simulink model "mpc_model_dual_module_tobecombined"  (R2019a)
settings: Solver=FixedStepAuto  StartTime=0.0  StopTime=Tfinal  RelTol=1e-3
values from neighbouring files (symbols this model uses):
  A = [-0.0285 -0.0014; -0.0371 -0.1476]    [model.m]
  DCLINK_Cap = 1000e-12    (= 1e-09)    [mpc_model_parameters.m]    (also in mpc_model_parameters_dual_module.m = 0.001)
  FluxPM = MeanInducedVoltagePeak/(2*pi*100)    [mpc_model_parameters.m]    (also in mpc_model_parameters_dual_module.m)
  Inertia = 1e-2    (= 0.01)    [mpc_model_parameters.m]    (also in mpc_model_parameters_dual_module.m)
  iqrated = Trated/(1.5*PolePairs*FluxPM)    [mpc_model_parameters.m]    (also in mpc_model_parameters_dual_module.m)
  Ls = 3.5e-3    (= 0.0035)    [MPC_id_iq.m]    (also in mpc_model_parameters.m = 0.00351; mpc_model_parameters_dual_module.m = 0.00343)
  M1_FaultTime = 0.25    [mpc_model_parameters_dual_module.m]
  M2_FaultTime = 20    [mpc_model_parameters_dual_module.m]
  MeanLd = (1/12)*(Module1Phase_A_Ld+Module1Phase_B_Ld+Module1Phase_C_Ld+     Module2Phase_A_Ld+Module2Phase_B_Ld+Module2Phase_C_Ld+     Module3Phase_A_Ld+Module3Phase_B_Ld+Module3Phase_C_Ld+     Module4Phase_A_Ld+Module4Phase_B_Ld+Module4Phase_C_Ld)    [mpc_model_parameters.m]    (also in mpc_model_parameters_dual_module.m)
  MeanLq = (1/12)*(Module1Phase_A_Lq+Module1Phase_B_Lq+Module1Phase_C_Lq+     Module2Phase_A_Lq+Module2Phase_B_Lq+Module2Phase_C_Lq+     Module3Phase_A_Lq+Module3Phase_B_Lq+Module3Phase_C_Lq+     Module4Phase_A_Lq+Module4Phase_B_Lq+Module4Phase_C_Lq)    [mpc_model_parameters.m]    (also in mpc_model_parameters_dual_module.m)
  PolePairs = 10    [mpc_model_parameters.m]    (also in mpc_model_parameters_dual_module.m)
  Rin = 1e-3    (= 0.001)    [mpc_model_parameters.m]    (also in mpc_model_parameters_dual_module.m)
  Rs = 0.531    [Loss_Distribution.m]    (also in MPC_id_iq.m; mpc_model_parameters.m = 0.321; mpc_model_parameters_dual_module.m = 0.539)
  Sampling_time = 1e-6    (= 1e-06)    [mpc_model_parameters.m]    (also in mpc_model_parameters_dual_module.m)
  SpeedRef1 = 50    [mpc_model_parameters.m]    (also in mpc_model_parameters_dual_module.m = 35)
  SpeedRef2 = 100    [mpc_model_parameters.m]    (also in mpc_model_parameters_dual_module.m = 35)
  SpeedRefUpdateTime = 0.25    [mpc_model_parameters.m]    (also in mpc_model_parameters_dual_module.m = 1.75)
  Tload1 = 5    [mpc_model_parameters.m]    (also in mpc_model_parameters_dual_module.m = 30)
  Tload2 = 10    [mpc_model_parameters.m]    (also in mpc_model_parameters_dual_module.m = 63.6619772368)
  TloadUpdateTime = 0.5    [mpc_model_parameters.m]    (also in mpc_model_parameters_dual_module.m)
  Vdc = 50    [mpc_model_parameters.m]    (also in mpc_model_parameters_dual_module.m = 40)
  Vin = Vdc + Rin*(Pout/Vdc)    (= 50.04)    [mpc_model_parameters.m]    (also in mpc_model_parameters_dual_module.m = 40.05)
  ViscousFriction = 1e-3    (= 0.001)    [mpc_model_parameters.m]    (also in mpc_model_parameters_dual_module.m)
undefined symbols (not defined in the file or in its folder): DiscIntNeverNeededParam
libraries: powerlib x24, dspswit3 x13, fl_lib x5, simulink x3, powerlib_meascontrol x3, nesl_utility x3, sdl_lib x1, dspsigops x1
(part 1 of 2)
settings Model: Creator=hakan  LastModifiedBy=hakan
settings SolverCC: ZeroCrossAlgorithm=Adaptive
settings DebuggingCC: IgnoredZcDiagnostic=none

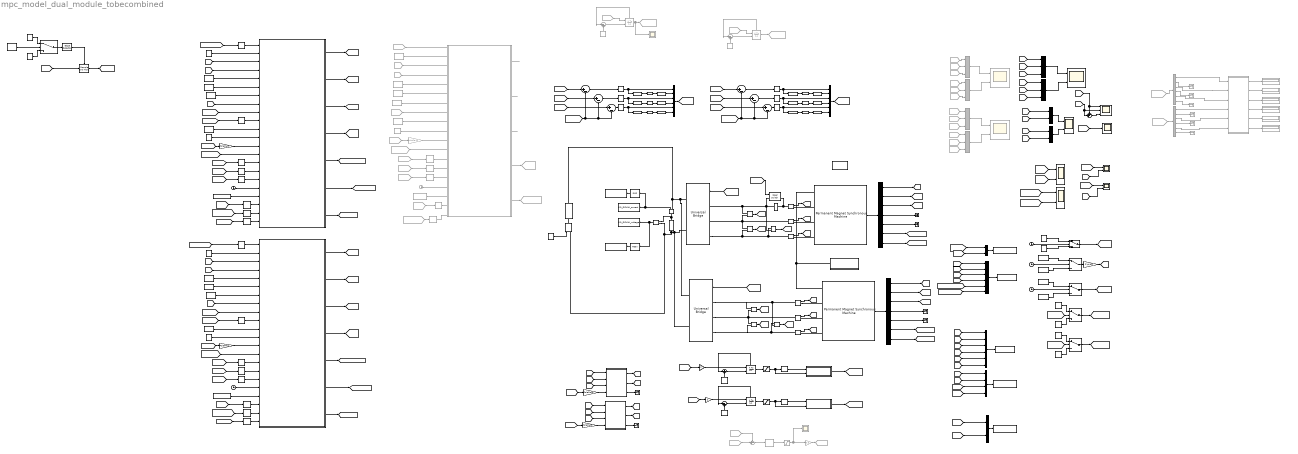
== system mpc_model_dual_module_tobecombined ==
  note: M1_thetam & M2_thetam will be the but they are seperated anyway
  A_DCLINK_current : ToWorkspace  VariableName=M1_DCLINK_current  SaveFormat=Structure With Time  SampleTime=-1
  A_DCLINK_current_rms : ToWorkspace  VariableName=M1_DCLINK_current_rms  SaveFormat=Structure With Time  SampleTime=-1
  A_DCLINK_voltage : ToWorkspace  VariableName=M1_DCLINK_voltage  SaveFormat=Structure With Time  SampleTime=-1
  A_DCLINK_voltage_mean : ToWorkspace  VariableName=M1_DCLINK_voltage_mean  SaveFormat=Structure With Time  SampleTime=-1
  Bus Creator : BusCreator  Inputs=6
  Bus Creator1 : BusCreator  Inputs=6
  Bus Creator{3,10..12} (4 alike) : BusCreator  Inputs=2
  Bus Creator2 : BusCreator  Inputs=4
  Bus Creator{4..7} (4 alike) : BusCreator  Commented=on  Inputs=3
  Bus Creator8 : BusCreator  Inputs=3
  Bus Creator9 : BusCreator  Inputs=3
  Bus Selector : BusSelector  OutputSignals=Electromagnetic torque Te (N*m),Rotor speed wm (rad/s),Rotor angle thetam (rad),Stator current is_q (A),Stator current is_d (A),Stator voltage Vs_q (V),Stator voltage Vs_d (V)
  Bus Selector1 : BusSelector  OutputSignals=Electromagnetic torque Te (N*m),Rotor speed wm (rad/s),Rotor angle thetam (rad),Stator current is_q (A),Stator current is_d (A),Stator voltage Vs_q (V),Stator voltage Vs_d (V)
  Clock{,1..2,4..5} (5 alike) : Clock
  Clock3 : Clock  Commented=on
  Compare To Zero : simulink/Logic and Bit Operations/Compare To Zero  relop===  OutDataTypeStr=boolean
  Compare To Zero1 : simulink/Logic and Bit Operations/Compare To Zero  relop===  OutDataTypeStr=boolean
  Constant : Constant  Value=Vin
  Constant1 : Constant  Commented=on  Value=1.04
  Constant10 : Constant  Value=SpeedRef1
  Constant11 : Constant  Value=SpeedRef2
  Constant12 : Constant  Value=Tload2
  Constant13 : Constant  Value=M2_FaultTime
  Constant14 : Constant  Value=Ls
  Constant{4,15,22,27,29,36} (6 alike) : Constant  Value=0
  Constant{16,23,30,37} (4 alike) : Constant
  Constant17 : Constant  Commented=on  Value=M1_FaultTime
  Constant18 : Constant  Value=Rs
  Constant19 : Constant  Value=PolePairs
  Constant2 : Constant  Commented=on  Value=0
  Constant20 : Constant  Value=FluxPM
  Constant21 : Constant  Value=Vdc
  Constant24 : Constant  Value=1.02
  Constant25 : Constant  Value=1.02
  Constant26 : Constant  Commented=on  Value=1.04
  Constant28 : Constant  Value=M1_FaultTime
  Constant3 : Constant  Commented=on  Value=Ls
  Constant31 : Constant  Value=Ls
  Constant32 : Constant  Value=Rs
  Constant33 : Constant  Value=PolePairs
  Constant34 : Constant  Value=FluxPM
  Constant35 : Constant  Value=Vdc
  Constant5 : Constant  Commented=on  Value=Rs
  Constant6 : Constant  Commented=on  Value=PolePairs
  Constant7 : Constant  Commented=on  Value=FluxPM
  Constant8 : Constant  Value=Tload1
  Constant9 : Constant  Commented=on  Value=Vdc
  Controlled Voltage Source : powerlib/Electrical Sources/Controlled Voltage Source  Initialize=on  Source_Type=DC  Amplitude=0  Phase=0  Frequency=0  Measurements=None
      settings: SourceProductName=Simscape Electrical
  Current Measurement{,1..6} (7 alike) : powerlib/Measurements/Current Measurement  PhasorSimulation=off  OutputType=Complex  PSBequivalent=0
      settings: SourceProductName=Simscape Electrical
  DCLINK_Cap : powerlib/Elements/Series RLC Branch  LConnTagsString=__new0  RConnTagsString=__new0  BranchType=C  Resistance=1  Inductance=1e-3  SetiL0=off  InitialCurrent=0  Capacitance=DCLINK_Cap  Setx0=on  InitialVoltage=Vin  Measurements=None
      settings: SourceProductName=Simscape Electrical
  Data Type Conversion{1,3,5,12,14,16} (6 alike) : DataTypeConversion  OutDataTypeStr=boolean
  Data Type Conversion{2,4,6,13,15,17} (6 alike) : DataTypeConversion  OutDataTypeStr=double
  Delay{,2..10,15..20} (16 alike) : Delay  DelayLength=1
  Delay{1,11..14} (5 alike) : Delay  Commented=on  DelayLength=1
  Demux2 : Demux  Commented=on  Outputs=6
  Demux3 : Demux  Commented=on  Outputs=6
  Discrete-Time Integrator : DiscreteIntegrator  Commented=on  ExternalReset=falling  SampleTime=-1  ShowStatePort=on  ICPrevOutput=DiscIntNeverNeededParam  ICPrevScaledInput=DiscIntNeverNeededParam
  Discrete-Time Integrator1 : DiscreteIntegrator  Commented=on  ExternalReset=falling  SampleTime=-1  ShowStatePort=on  ICPrevOutput=DiscIntNeverNeededParam  ICPrevScaledInput=DiscIntNeverNeededParam
  Discrete-Time Integrator2 : DiscreteIntegrator  ExternalReset=falling  SampleTime=Sampling_time  UpperSaturationLimit=1  LowerSaturationLimit=0  ShowStatePort=on  ICPrevOutput=DiscIntNeverNeededParam  ICPrevScaledInput=DiscIntNeverNeededParam
  Discrete-Time Integrator3 : DiscreteIntegrator  ExternalReset=falling  SampleTime=Sampling_time  UpperSaturationLimit=1  LowerSaturationLimit=0  ShowStatePort=on  ICPrevOutput=DiscIntNeverNeededParam  ICPrevScaledInput=DiscIntNeverNeededParam
  Display{1..6} (6 alike) : Display  Commented=on
  Edge Detector3 : dspswit3/Edge Detector  InputProcessing=Columns as channels (frame based)
      settings: SourceProductName=DSP System Toolbox  SourceProductBaseCode=DS
  From10 : From  Commented=on  GotoTag=M1_Vbc
  From100 : From  Commented=on  GotoTag=wref
  From101 : From  Commented=on  GotoTag=M1_wmech
  From11 : From  Commented=on  GotoTag=M1_Vca
  From13 : From  Commented=on  GotoTag=M1_IqRipplePrediction
  From14 : From  Commented=on  GotoTag=M1_wmech
  From17 : From  Commented=on  GotoTag=M1_thetam
  From22 : From  Commented=on  GotoTag=M1_fsw_out
  From23 : From  Commented=on  GotoTag=M1_iqref
  From28 : From  Commented=on  GotoTag=M1_switching_pulse
  From29 : From  Commented=on  GotoTag=M1_iqs
  From32 : From  Commented=on  GotoTag=M1_va_1
  From33 : From  Commented=on  GotoTag=M1_vb_1
  From34 : From  Commented=on  GotoTag=M1_vc_1
  From42 : From  Commented=on  GotoTag=M1_mpcgate
  From58 : From  Commented=on  GotoTag=M2_Vbc
  From59 : From  Commented=on  GotoTag=M2_Vca
  From6 : From  Commented=on  GotoTag=M1_mpcgate
  From60 : From  Commented=on  GotoTag=M2_Vab
  From61 : From  Commented=on  GotoTag=M2_va_1
  From62 : From  Commented=on  GotoTag=M2_vb_1
  From63 : From  Commented=on  GotoTag=M2_vc_1
  From7 : From  Commented=on  GotoTag=M1_ids
  From77 : From  Commented=on  GotoTag=M1_fsw_out
  From78 : From  Commented=on  GotoTag=M1_DutyC
  From79 : From  Commented=on  GotoTag=M1_DutyB
  From80 : From  Commented=on  GotoTag=M1_DutyA
  From84 : From  Commented=on  GotoTag=M2_fsw_out
  From9 : From  Commented=on  GotoTag=M1_Vab
  Gain{,2,4,6} (4 alike) : Gain  Gain=PolePairs
  Gain1 : Gain  Gain=2*pi/60
  Gain3 : Gain  Commented=on  Gain=PolePairs
  Gain5 : Gain  Commented=on  Gain=0.5
  Gain7 : Gain  Gain=2
  Gain8 : Gain  Gain=2
  Goto13 : Goto  Commented=on  GotoTag=M1_IqRipplePrediction
  Goto35 : Goto  Commented=on  GotoTag=M2_CarrierSignal
  Goto36 : Goto  Commented=on  GotoTag=M1_fsw_out
  Goto39 : Goto  Commented=on  GotoTag=M1_CarrierSignal
  Goto46 : Goto  Commented=on  GotoTag=M2_iqref
  Ideal Switch : powerlib/Power Electronics/Ideal Switch  Ron=0.001  Lon=0  IC=0  Rs=1e5  Cs=inf  Measurements=on
      settings: SourceProductName=Simscape Electrical
  Inverter1 : powerlib/Power Electronics/Universal Bridge  Arms=3  SnubberResistance=1e5  SnubberCapacitance=inf  Device=IGBT / Diodes  Ron=0.65e-3  Lon=0  ForwardVoltages="[  0  0  ]"  ForwardVoltage=0  GTOparameters=[ 10e-6 , 20e-6 ]  IGBTparameters=[ 1e-6 , 2e-6 ]  Measurements=All voltages and currents  Measurements_2=None  converterType=Rectifier
      settings: SourceProductName=Simscape Electrical
  Inverter2 : powerlib/Power Electronics/Universal Bridge  Arms=3  SnubberResistance=1e5  SnubberCapacitance=inf  Device=IGBT / Diodes  Ron=0.65e-3  Lon=0  ForwardVoltages="[  0  0  ]"  ForwardVoltage=0  GTOparameters=[ 10e-6 , 20e-6 ]  IGBTparameters=[ 1e-6 , 2e-6 ]  Measurements=All voltages and currents  Measurements_2=None  converterType=Rectifier
      settings: SourceProductName=Simscape Electrical
  Logical Operator{1..3,6..8} (6 alike) : Logic  Operator=NOT  AllPortsSameDT=off  OutDataTypeStr=boolean
  M1_prediction : MATLAB Function  Commented=on  TreatAsAtomicUnit=on
  MATLAB Function1 : MATLAB Function  TreatAsAtomicUnit=on
  MATLAB Function2 : MATLAB Function  TreatAsAtomicUnit=on
  Mean : powerlib_meascontrol/Measurements/Mean  Freq=THD_mean_frequency  Vinit=0  Ts=Sampling_time
      settings: SourceProductName=Simscape Electrical
  Mean Switching Frequency : Subsystem  Commented=on
  Mechanical Subsystem : Subsystem
  Mux1 : Mux  Inputs=6
  Mux4 : Mux  Inputs=6
  PID Controller2 : simulink/Continuous/PID Controller  Commented=on  Controller=PID  Form=Parallel  TimeDomain=Continuous-time  SampleTime=-1  IntegratorMethod=Forward Euler  FilterMethod=Forward Euler  ControllerParametersSource=internal  P=1  I=10  D=0  UseFilter=on  N=100  TunerSelectOption=Transfer Function Based (PID Tuner App)  InitialConditionSource=internal  InitialConditionForIntegrator=0  InitialConditionForFilter=0  DifferentiatorICPrevScaledInput=0  ExternalReset=none  TrackingMode=off  Kt=1  LimitOutput=off  UpperSaturationLimit=inf  LowerSaturationLimit=-inf  LinearizeAsGain=on  AntiWindupMode=none  Kb=1  POutMin=[]  POutMax=[]  IOutMin=[]  IOutMax=[]  DOutMin=[]  DOutMax=[]  NOutMin=[]  NOutMax=[]  SumOutMin=[]  SumOutMax=[]  SaturationOutMin=[]  SaturationOutMax=[]  PParamMin=[]  PParamMax=[]  IParamMin=[]  IParamMax=[]  DParamMin=[]  DParamMax=[]  NParamMin=[]  NParamMax=[]  KbParamMin=[]  KbParamMax=[]  KtParamMin=[]  KtParamMax=[]  KbOutMin=[]  KbOutMax=[]  KtOutMin=[]  KtOutMax=[]  IntegratorOutMin=[]  IntegratorOutMax=[]  FilterOutMin=[]  FilterOutMax=[]  SumI1OutMin=[]  SumI1OutMax=[]  SumI2OutMin=[]  SumI2OutMax=[]  SumI3OutMin=[]  SumI3OutMax=[]  SumI4OutMin=[]  SumI4OutMax=[]  SumDOutMin=[]  SumDOutMax=[]  DifferentiatorOutMin=[]  DifferentiatorOutMax=[]  FilterDiffOutCoefMin=[]  FilterDiffOutCoefMax=[]  ReciprocalOutMin=[]  ReciprocalOutMax=[]  SumDenOutMin=[]  SumDenOutMax=[]  SumNumOutMin=[]  SumNumOutMax=[]  DivideOutMin=[]  DivideOutMax=[]  IntegratorContinuousStateAttributes=''  IntegratorStateMustResolveToSignalObject=off  IntegratorRTWStateStorageClass=Auto  FilterContinuousStateAttributes=''  FilterStateMustResolveToSignalObject=off  FilterRTWStateStorageClass=Auto  ParallelPVariant=InternalParameters  IdealPVariant=Disabled  IVariant=InternalParameters  DVariant=InternalParameters  IntegratorVariant=Continuous  SatVariant=Disabled  AWVariant=Passthrough  PCopyVariant=Disabled  TRVariant=Disabled  FdbkBlocksVariant=Forward  IdealPFdbkVariant=Disabled  SatFdbkVariant=Disabled  DerivativeFilterVariant=ContFilter  NVariant=InternalParameters  NCopyVariant=Disabled  FilterICVariant=InternalICsFilter  IntegratorICVariant=InternalICs  ExternalResetVariant=Disabled  TRSumVariant=Passthrough  SumFdbkVariant=Disabled  SumVariant=Sum_PID
  Permanent Magnet Synchronous Machine : powerlib/Machines/Permanent Magnet Synchronous Machine  NbPhases=3  FluxDistribution=Sinusoidal  RotorType=Round  MechanicalLoad=Mechanical rotational port  PresetModel=No  ShowDetailedParameters=on  MeasurementBus=off  Resistance=Rs  Inductance=8.5e-3  dqInductances=[MeanLd,MeanLq]  La=Ls  MachineConstant=Voltage Constant (V_peak L-L / krpm)  Flux=0.18074  VoltageCst=VoltageConstant  TorqueCst=2.7111  Flat=120  Mechanical=[Inertia ViscousFriction PolePairs 0]  PolePairs=4  InitialConditions=[0,0, 0,0]  InitialConditions5ph=[0 0 0 0 0 0]  TsPowergui=0  TsBlock=-1  RefAngle=90 degrees behind phase A axis (modified Park)
  Permanent Magnet Synchronous Machine1 : powerlib/Machines/Permanent Magnet Synchronous Machine  NbPhases=3  FluxDistribution=Sinusoidal  RotorType=Round  MechanicalLoad=Mechanical rotational port  PresetModel=No  ShowDetailedParameters=on  MeasurementBus=off  Resistance=Rs  Inductance=8.5e-3  dqInductances=[MeanLd,MeanLq]  La=Ls  MachineConstant=Voltage Constant (V_peak L-L / krpm)  Flux=0.18074  VoltageCst=VoltageConstant  TorqueCst=2.7111  Flat=120  Mechanical=[Inertia ViscousFriction PolePairs 0]  PolePairs=4  InitialConditions=[0,0, 0,0]  InitialConditions5ph=[0 0 0 0 0 0]  TsPowergui=0  TsBlock=-1  RefAngle=90 degrees behind phase A axis (modified Park)
  RMS1 : powerlib_meascontrol/Measurements/RMS  TrueRMS=on  Freq=Load_Nominal_Freq  RMSInit=10  Ts=Sampling_time
      settings: SourceProductName=Simscape Electrical
  Relay{,1..5} (6 alike) : Relay
  Rin : powerlib/Elements/Series RLC Branch  LConnTagsString=__new0  RConnTagsString=__new0  BranchType=R  Resistance=Rin  Inductance=1e-3  SetiL0=off  InitialCurrent=0  Capacitance=1000e-6  Setx0=off  InitialVoltage=0  Measurements=None
      settings: SourceProductName=Simscape Electrical
  Sample and Hold : dspsigops/Sample and Hold  trig=Rising edge  initCond=0  latchinput=off
  Saturation : Saturate  Commented=on  UpperLimit=4*iqrated  LowerLimit=-4*iqrated  LinearizeAsGain=off
  Saturation1 : Saturate  UpperLimit=1  LowerLimit=0
  Saturation2 : Saturate  UpperLimit=1  LowerLimit=0
  Sawtooth Generator : powerlib_meascontrol/Pulse & Signal Generators/Sawtooth Generator  Freq=100  Phase=180  Ts=0
      settings: SourceProductName=Simscape Electrical
  Scope : Scope  NumInputPorts=3
  Scope1 : Scope
  Scope{5..10} (6 alike) : Scope  NumInputPorts=2
  Scope12 : Scope  Commented=on
  Scope2 : Scope  Commented=on  NumInputPorts=2
  Scope3 : Scope  Commented=on
  Scope4 : Scope  Commented=on  NumInputPorts=2
  Series RLC Branch : powerlib/Elements/Series RLC Branch  LConnTagsString=__new0  RConnTagsString=__new0  BranchType=R  Resistance=5000  Inductance=1e-3  SetiL0=off  InitialCurrent=0  Capacitance=1e-6  Setx0=off  InitialVoltage=0  Measurements=None
      settings: SourceProductName=Simscape Electrical
  Sum : Sum  Commented=on  Inputs=-+|
  Sum1 : Sum  Inputs=++|
  Sum10 : Sum  Inputs=|-+
  Sum12 : Sum  Inputs=|-+
  Sum{2,4..6,8..9} (6 alike) : Sum  Inputs=|+-
  Sum3 : Sum  Commented=on  Inputs=|-+
  Sum7 : Sum  Commented=on  Inputs=|-+
  Switch : Switch  Criteria=u2 > Threshold  Threshold=SpeedRefUpdateTime
  Switch1 : Switch  Criteria=u2 > Threshold  Threshold=TloadUpdateTime
  Switch2 : Switch  Criteria=u2 ~= 0
  Switch3 : Switch  Criteria=u2 > Threshold  Threshold=M1_FaultTime
  Switch4 : Switch  Criteria=u2 ~= 0
  Switch5 : Switch  Threshold=0.99
  Terminator{,4..8} (6 alike) : Terminator
  Terminator{1,10..14} (6 alike) : Terminator  Commented=on
  To Workspace1 : ToWorkspace  VariableName=Simout_PhaseCurrents_abc  SaveFormat=Timeseries  SampleTime=-1
  To Workspace2 : ToWorkspace  VariableName=Simout_PhaseCurrents_dq  SaveFormat=Timeseries  SampleTime=-1
  To Workspace3 : ToWorkspace  VariableName=Simout_TorqueSpeedMeas  SaveFormat=Timeseries  SampleTime=-1
  To Workspace4 : ToWorkspace  VariableName=Simout_TorqueSpeedRef  SaveFormat=Timeseries  SampleTime=-1
  To Workspace5 : ToWorkspace  VariableName=Simout_Fsw  SaveFormat=Timeseries  SampleTime=-1
  Voltage Measurement{,1..6} (7 alike) : powerlib/Measurements/Voltage Measurement  PhasorSimulation=off  OutputType=Complex  PSBequivalent=0
      settings: SourceProductName=Simscape Electrical
  module 1 abc to dq0 : MATLAB Function  TreatAsAtomicUnit=on
  module 2 abc to dq0 : MATLAB Function  TreatAsAtomicUnit=on
  powergui : powerlib/powergui  Priority=1  SimulationMode=Discrete  SampleTime=Sampling_time  frequency=60  Iterations=50  frequencyindice=0  Pbase=100e6  ErrMax=1e-4  UnitsV=kV  UnitsW=MW  buscounter=0  FunctionMessages=off  echomessages=off  EnableUseOfTLC=off  CurrentSourceSwitches=off  DisableSnubberDevices=off  DisableRonSwitches=off  DisableVfSwitches=off  DisplayEquations=off  AutomaticDiscreteSolvers=off  SolverType=Tustin/Backward Euler (TBE)  Interpol=off  ExternalGateDelay=off  methode=off  Ts=100  x0status=blocks  SPID=on  SwTol=0  HookPort=off  NonlinearTolerance=0  nMaxIteration=15  ContinueOnMaxIteration=off  RestoreLinks=warning  ResistiveCurrentMeasurement=off  Frange=[0:2:500]  Ylog=off  Xlog=on  ShowGrid=off  save=off  variable=ZData  structure=0  ZoomFFT=off  StartTime=0.0  cycles=1  DisplayStyle=1  fundamental=60  FreqAxis=off  MaxFrequency=1000  frequencyindicesteady=1  RmsSteady=1  display=off
      settings: SourceProductName=Simscape Electrical
  prediction : MATLAB Function  TreatAsAtomicUnit=on
  prediction1 : MATLAB Function  TreatAsAtomicUnit=on
  wires:
  Voltage Measurement3/1 -> Mean/1, A_DCLINK_voltage/1
  RMS1/1 -> A_DCLINK_current_rms/1
  Constant/1 -> Controlled Voltage Source/1
  Mean/1 -> A_DCLINK_voltage_mean/1
  Current Measurement/1 -> RMS1/1, A_DCLINK_current/1
  Permanent Magnet Synchronous Machine/1 -> Bus Selector/1
  Bus Selector/1 -> [M1_Te]  "<Electromagnetic torque Te (N*m)>"
  Bus Selector/2 -> [M1_wmech]  "<Rotor speed wm (rad/s)>"
  Current Measurement1/1 -> [M1_Ia]
  Current Measurement2/1 -> [M1_Ib]
  Current Measurement3/1 -> [M1_Ic]
  Bus Selector/3 -> [M1_thetam]  "<Rotor angle thetam (rad)>"
  [M1_thetam] -> Gain/1
  [M1_Ia] -> module 1 abc to dq0/1(ias)
  [M1_Ib] -> module 1 abc to dq0/2(ibs)
  [M1_Ic] -> module 1 abc to dq0/3(ics)
  Gain/1 -> module 1 abc to dq0/4(ref_frame_position)
  Bus Selector/4 -> Terminator4/1  "<Stator current is_q (A)>"
  Bus Selector/5 -> Terminator5/1  "<Stator current is_d (A)>"
  module 1 abc to dq0/2(iqs) -> [M1_iqs]
  module 1 abc to dq0/1(ids) -> [M1_ids]
  module 1 abc to dq0/3(i0) -> Terminator/1
  Voltage Measurement/1 -> [M1_Vab]
  Voltage Measurement1/1 -> [M1_Vbc]
  Voltage Measurement2/1 -> [M1_Vca]
  Bus Selector/6 -> [M1_vsq_actual]  "<Stator voltage Vs_q (V)>"
  Bus Selector/7 -> [M1_vsd_actual]  "<Stator voltage Vs_d (V)>"
  [M1_mpcgate] -> Inverter1/1
  [M1_iqs] -> Bus Creator1/2  "M1_iqs"
  [M1_ids] -> Bus Creator1/1  "M1_ids"
  Constant10/1 -> Switch/3
  Constant11/1 -> Switch/1
  Switch/1 -> Gain1/1
  Clock/1 -> Switch/2
  Clock1/1 -> Switch1/2
  Constant12/1 -> Switch1/1
  Constant8/1 -> Switch1/3
  Switch1/1 -> [Combined_Tload]
  Bus Creator/1 -> To Workspace1/1  "Iabc"
  Bus Creator1/1 -> To Workspace2/1  "Idq"
  Bus Creator2/1 -> To Workspace3/1
  Gain1/1 -> [wref]
  [Combined_Tload] -> Bus Creator3/1  "Combined_Tload"
  [wref] -> Bus Creator3/2  "wref"
  Bus Creator3/1 -> To Workspace4/1
  [M1_Ib] -> Bus Creator/2  "M1_Ib"
  [M1_Ia] -> Bus Creator/1  "M1_Ia"
  [M1_Ic] -> Bus Creator/3  "M1_Ic"
  [M1_iqs] -> Bus Creator10/1  "M1_iqs"
  [M1_ids] -> Bus Creator10/2  "M1_ids"
  [M1_Te] -> Bus Creator2/1  "M1_Te"
  [M1_Te] -> Sum1/1, Scope/1  "M1_Te"
  [M1_wmech] -> Scope1/1  "M1_wmech"
  [M1_FaultTrig] -> Ideal Switch/1
  Constant16/1 -> Switch3/3
  Clock2/1 -> Switch3/2
  Constant15/1 -> Switch3/1
  Switch3/1 -> [M1_FaultTrig]
  [M1_wmech] -> Bus Creator2/3  "M1_wmech"
  [M2_Te] -> Bus Creator2/2  "M2_Te"
  Bus Selector1/7 -> [M2_vsd_actual]  "<Stator voltage Vs_d (V)>"
  Bus Selector1/6 -> [M2_vsq_actual]  "<Stator voltage Vs_q (V)>"
  Bus Selector1/5 -> Terminator7/1  "<Stator current is_d (A)>"
  Bus Selector1/4 -> Terminator6/1  "<Stator current is_q (A)>"
  Bus Selector1/3 -> [M2_thetam]  "<Rotor angle thetam (rad)>"
  Bus Selector1/2 -> [M2_wmech]  "<Rotor speed wm (rad/s)>"
  Bus Selector1/1 -> [M2_Te]  "<Electromagnetic torque Te (N*m)>"
  Permanent Magnet Synchronous Machine1/1 -> Bus Selector1/1
  module 2 abc to dq0/3(i0) -> Terminator8/1
  module 2 abc to dq0/1(ids) -> [M2_ids]
  module 2 abc to dq0/2(iqs) -> [M2_iqs]
  Gain2/1 -> module 2 abc to dq0/4(ref_frame_position)
  [M2_Ic] -> module 2 abc to dq0/3(ics)
  [M2_Ib] -> module 2 abc to dq0/2(ibs)
  [M2_Ia] -> module 2 abc to dq0/1(ias)
  [M2_thetam] -> Gain2/1
  Current Measurement4/1 -> [M2_Ia]
  Current Measurement5/1 -> [M2_Ib]
  Current Measurement6/1 -> [M2_Ic]
  Voltage Measurement5/1 -> [M2_Vbc]
  Voltage Measurement4/1 -> [M2_Vab]
  Voltage Measurement6/1 -> [M2_Vca]
  [M2_wmech] -> Bus Creator2/4  "M2_wmech"
  [M2_ids] -> Bus Creator1/3  "M2_ids"
  [M2_iqs] -> Bus Creator1/4  "M2_iqs"
  [M2_Ic] -> Bus Creator/6  "M2_Ic"
  [M2_Ia] -> Bus Creator/4  "M2_Ia"
  [M2_Ib] -> Bus Creator/5  "M2_Ib"
  [M2_Te] -> Sum1/2, Scope/2  "M2_Te"
  From10/1 -> Bus Creator5/2
  From9/1 -> Bus Creator5/1
  From11/1 -> Bus Creator5/3
  From59/1 -> Bus Creator4/3
  From60/1 -> Bus Creator4/1
  From58/1 -> Bus Creator4/2
  Bus Creator4/1 -> Scope2/2  "M2_Vlinetoline_abc"
  Bus Creator5/1 -> Scope2/1  "M1_Vlinetoline_abc"
  Bus Creator7/1 -> Scope4/1  "M1_gate"
  Bus Creator6/1 -> Scope4/2  "M2_gate"
  From62/1 -> Bus Creator6/2
  From61/1 -> Bus Creator6/1
  From63/1 -> Bus Creator6/3
  From34/1 -> Bus Creator7/3
  From33/1 -> Bus Creator7/2
  From32/1 -> Bus Creator7/1
  Bus Creator9/1 -> Scope5/1  "M1_Iabc"
  Bus Creator8/1 -> Scope5/2  "M2_Iabc"
  [M2_Ib] -> Bus Creator8/2
  [M2_Ia] -> Bus Creator8/1
  [M2_Ic] -> Bus Creator8/3
  [M1_Ic] -> Bus Creator9/3
  [M1_Ia] -> Bus Creator9/1
  [M1_Ib] -> Bus Creator9/2
  Bus Creator10/1 -> Scope8/1  "M1_iqds"
  [M2_ids] -> Bus Creator11/2  "M2_ids"
  [M2_iqs] -> Bus Creator11/1  "M2_iqs"
  Bus Creator11/1 -> Scope8/2  "M2_iqds"
  Demux2/1 -> Mean Switching Frequency/1(In1)
  Demux2/3 -> Mean Switching Frequency/2(In2)
  Demux2/5 -> Mean Switching Frequency/3(In3)
  Mean Switching Frequency/1(Out1) -> Display2/1
  Mean Switching Frequency/2(Out2) -> Display1/1
  Mean Switching Frequency/3(Out3) -> Display3/1
  Mean Switching Frequency/4(Out4) -> Display5/1
  Mean Switching Frequency/5(Out5) -> Display4/1
  Mean Switching Frequency/6(Out6) -> Display6/1
  [M2_mpcgate] -> Inverter2/1
  Sum1/1 -> Scope/3
  M1_prediction/5(IqRipplePrediction) -> Goto13/1
  Delay14/1 -> M1_prediction/15(DutyC_prev)
  Constant6/1 -> M1_prediction/7(PolePairs)
  From78/1 -> Delay14/1
  Delay1/1 -> M1_prediction/19(IqRipplePrediction_prev)
  Constant7/1 -> M1_prediction/9(FluxPM)
  Constant9/1 -> M1_prediction/10(Vdc)
  Delay13/1 -> M1_prediction/14(DutyB_prev)
  From13/1 -> Delay1/1
  Delay12/1 -> M1_prediction/13(DutyA_prev)
  M1_prediction/2(DutyB) -> ?
  Clock3/1 -> M1_prediction/16(SimulationClock)
  From79/1 -> Delay13/1
  M1_prediction/3(DutyC) -> ?
  M1_prediction/1(DutyA) -> ?
  From29/1 -> M1_prediction/4(IqMeasured)
  Constant17/1 -> M1_prediction/17(FaultOccuranceTime)
  From14/1 -> M1_prediction/8(ShaftAngularSpeed)
  From28/1 -> M1_prediction/12(InterruptPulse)
  Gain3/1 -> M1_prediction/11(ElectricalAngle)
  M1_prediction/4(FswSelected) -> Goto36/1
  From17/1 -> Gain3/1
  Delay11/1 -> M1_prediction/18(FswSelected_prev)
  Constant3/1 -> M1_prediction/5(Ls)
  From7/1 -> M1_prediction/3(IdMeasured)
  From22/1 -> Delay11/1
  Constant2/1 -> M1_prediction/2(idref)
  Constant5/1 -> M1_prediction/6(Rs)
  From80/1 -> Delay12/1
  Sum3/1 -> Discrete-Time Integrator/2
  Discrete-Time Integrator/State -> Sum3/1
  Discrete-Time Integrator/1 -> Goto39/1
  From77/1 -> Discrete-Time Integrator/1
  Constant26/1 -> Sum3/2
  Relay/1 -> Mux4/1, Data Type Conversion14/1
  Mux4/1 -> [M1_mpcgate]
  Sum5/1 -> Relay1/1
  Logical Operator8/1 -> Data Type Conversion13/1
  Logical Operator7/1 -> Data Type Conversion17/1
  [M1_DutyB] -> Sum5/1
  Sum2/1 -> Relay/1
  Data Type Conversion15/1 -> Mux4/2
  Sum6/1 -> Relay2/1
  Logical Operator6/1 -> Data Type Conversion15/1
  Data Type Conversion12/1 -> Logical Operator8/1
  Relay1/1 -> Data Type Conversion16/1, Mux4/3
  Data Type Conversion13/1 -> Mux4/6
  [M1_CarrierSignal] -> Sum2/2, Sum5/2, Sum6/2
  Data Type Conversion14/1 -> Logical Operator6/1
  [M1_DutyC] -> Sum6/1
  Relay2/1 -> Data Type Conversion12/1, Mux4/5
  [M1_DutyA] -> Sum2/1
  Data Type Conversion16/1 -> Logical Operator7/1
  Data Type Conversion17/1 -> Mux4/4
  Constant29/1 -> Switch4/1
  Constant30/1 -> Switch4/3
  Switch4/1 -> [M1_switching_pulse]
  [M1_CarrierSignal] -> Switch4/2
  Data Type Conversion6/1 -> Mux1/4
  Data Type Conversion5/1 -> Logical Operator2/1
  [M2_DutyA] -> Sum4/1
  Relay5/1 -> Mux1/5, Data Type Conversion1/1
  [M2_DutyC] -> Sum9/1
  Data Type Conversion3/1 -> Logical Operator1/1
  [M2_CarrierSignal] -> Sum9/2, Sum8/2, Sum4/2
  Data Type Conversion2/1 -> Mux1/6
  Relay4/1 -> Mux1/3, Data Type Conversion5/1
  Data Type Conversion1/1 -> Logical Operator3/1
  Logical Operator1/1 -> Data Type Conversion4/1
  Sum9/1 -> Relay5/1
  Data Type Conversion4/1 -> Mux1/2
  Sum4/1 -> Relay3/1
  [M2_DutyB] -> Sum8/1
  Logical Operator2/1 -> Data Type Conversion6/1
  Logical Operator3/1 -> Data Type Conversion2/1
  Sum8/1 -> Relay4/1
  Mux1/1 -> [M2_mpcgate]
  Relay3/1 -> Data Type Conversion3/1, Mux1/1
  Constant1/1 -> Sum7/2
  From84/1 -> Discrete-Time Integrator1/1
  Discrete-Time Integrator1/1 -> Scope12/1, Goto35/1
  Discrete-Time Integrator1/State -> Sum7/1
  Sum7/1 -> Discrete-Time Integrator1/2
  [M2_CarrierSignal] -> Switch2/2
  Switch2/1 -> [M2_switching_pulse]
  Constant23/1 -> Switch2/3
  Constant22/1 -> Switch2/1
  [M1_fsw_out] -> Scope6/1  "M1_fsw"
  [M2_fsw_out] -> Scope6/2  "M2_fsw"
  [M1_IqRipplePrediction] -> Scope7/1  "M1_iqripple"
  [M2_IqRipplePrediction] -> Scope7/2  "M2_iqripple"
  From23/1 -> M1_prediction/1(iqref)
  PID Controller2/1 -> Saturation/1
  Sum/1 -> PID Controller2/1
  From100/1 -> Sum/2
  From101/1 -> Sum/1
  Saturation/1 -> Scope3/1, Gain5/1
  Gain5/1 -> Goto46/1
  Demux2/4 -> Terminator10/1
  Demux2/6 -> Terminator1/1
  From42/1 -> Demux2/1
  Demux2/2 -> Terminator11/1
  Demux3/2 -> Terminator14/1
  From6/1 -> Demux3/1
  Demux3/6 -> Terminator12/1
  Demux3/4 -> Terminator13/1
  Demux3/5 -> Mean Switching Frequency/6(In6)
  Demux3/3 -> Mean Switching Frequency/5(In5)
  Demux3/1 -> Mean Switching Frequency/4(In4)
  Discrete-Time Integrator2/1 -> Saturation1/1
  Sum10/1 -> Discrete-Time Integrator2/2
  Compare To Zero/1 -> MATLAB Function1/1(pulse)
  MATLAB Function1/1(outputwave) -> [M1_CarrierSignal]
  [M1_fsw_out] -> Gain8/1
  Saturation1/1 -> MATLAB Function1/2(inputwave), Compare To Zero/1
  Discrete-Time Integrator2/State -> Sum10/1
  Constant24/1 -> Sum10/2
  Constant25/1 -> Sum12/2
  Discrete-Time Integrator3/State -> Sum12/1
  Saturation2/1 -> Compare To Zero1/1, MATLAB Function2/2(inputwave)
  [M2_fsw_out] -> Gain7/1
  MATLAB Function2/1(outputwave) -> [M2_CarrierSignal]
  Compare To Zero1/1 -> MATLAB Function2/1(pulse)
  Sum12/1 -> Discrete-Time Integrator3/2
  Discrete-Time Integrator3/1 -> Saturation2/1
  Gain7/1 -> Discrete-Time Integrator3/1
  Gain8/1 -> Discrete-Time Integrator2/1
  Bus Creator12/1 -> To Workspace5/1
  [M2_fsw_out] -> Bus Creator12/2  "M2_fsw_out"
  [M1_fsw_out] -> Bus Creator12/1  "M1_fsw_out"
  [M1_IqRipplePrediction] -> Bus Creator1/5  "M1_iqripple"
  [M2_IqRipplePrediction] -> Bus Creator1/6  "M2_iqripple"
  [M2_iqref] -> Scope10/1  "M2_iqref"
  [M2_iqs] -> Scope10/2  "M2_iqs"
  [M1_iqref] -> Scope9/1  "M1_iqref"
  [M1_iqs] -> Scope9/2  "M1_iqs"
  [M1_ids] -> prediction/3(M1_IdMeasured)
  [M1_DutyC] -> Delay15/1
  Delay7/1 -> prediction/21(M1_IqRipplePrediction_prev)
  [M1_iqs] -> prediction/4(M1_IqMeasured)
  [wmech_lowrate] -> Delay17/1
  Delay16/1 -> prediction/22(M1_Speed_Error_prev)
  prediction/1(M1_DutyA) -> [M1_DutyA]
  prediction/7(M1_Speed_Error) -> [M1_Speed_Error]
  Gain6/1 -> prediction/13(ElectricalAngle)
  [M1_Speed_Error] -> Delay16/1
  Delay/1 -> prediction/1(M1_iqref_prev)
  [wref] -> prediction/8(wref)
  [M1_DutyB] -> Delay10/1
  [M1_DutyA] -> Delay9/1
  Constant27/1 -> prediction/2(M1_idref)
  prediction/5(M1_IqRipplePrediction) -> [M1_IqRipplePrediction]
  Delay9/1 -> prediction/15(M1_DutyA_prev)
  prediction/2(M1_DutyB) -> [M1_DutyB]
  Constant31/1 -> prediction/5(Ls)
  Delay10/1 -> prediction/16(M1_DutyB_prev)
  prediction/3(M1_DutyC) -> [M1_DutyC]
  Constant28/1 -> prediction/19(M1_FaultOccuranceTime)
  [M1_IqRipplePrediction] -> Delay7/1
  Delay8/1 -> prediction/20(M1_FswSelected_prev)
  Delay15/1 -> prediction/17(M1_DutyC_prev)
  Clock5/1 -> prediction/18(SimulationClock)
  [M1_switching_pulse] -> prediction/14(M1_InterruptPulse)
  Constant33/1 -> prediction/7(PolePairs)
  Delay17/1 -> prediction/10(ShaftAngularSpeed_prev)
  [wmech_lowrate] -> prediction/9(ShaftAngularSpeed)
  [M1_thetam] -> Gain6/1
  Constant35/1 -> prediction/12(Vdc)
  Constant34/1 -> prediction/11(FluxPM)
  Constant32/1 -> prediction/6(Rs)
  [M1_fsw_out] -> Delay8/1
  prediction/4(M1_FswSelected) -> [M1_fsw_out]
  Switch5/1 -> Edge Detector3/1
  Constant36/1 -> Switch5/1
  Constant37/1 -> Switch5/3
  Sample and Hold/1 -> [wmech_lowrate]
  Sawtooth Generator/1 -> Switch5/2
  Edge Detector3/1 -> Sample and Hold/Trigger
  [M1_wmech] -> Sample and Hold/1
  prediction1/4(M2_FswSelected) -> [M2_fsw_out]
  [M2_fsw_out] -> Delay19/1
  Constant18/1 -> prediction1/6(Rs)
  Constant20/1 -> prediction1/11(FluxPM)
  Constant21/1 -> prediction1/12(Vdc)
  [M2_thetam] -> Gain4/1
  [wmech_lowrate] -> prediction1/9(ShaftAngularSpeed)
  Delay6/1 -> prediction1/10(ShaftAngularSpeed_prev)
  Constant19/1 -> prediction1/7(PolePairs)
  [M2_switching_pulse] -> prediction1/14(M2_InterruptPulse)
  Clock4/1 -> prediction1/18(SimulationClock)
  Delay4/1 -> prediction1/17(M2_DutyC_prev)
  Delay19/1 -> prediction1/20(M2_FswSelected_prev)
  [M2_IqRipplePrediction] -> Delay18/1
  Constant13/1 -> prediction1/19(M2_FaultOccuranceTime)
  prediction1/3(M2_DutyC) -> [M2_DutyC]
  Delay3/1 -> prediction1/16(M2_DutyB_prev)
  Constant14/1 -> prediction1/5(Ls)
  prediction1/2(M2_DutyB) -> [M2_DutyB]
  Delay20/1 -> prediction1/15(M2_DutyA_prev)
  prediction1/5(M2_IqRipplePrediction) -> [M2_IqRipplePrediction]
  Constant4/1 -> prediction1/2(M2_idref)
  [M2_DutyA] -> Delay20/1
  [M2_DutyB] -> Delay3/1
  [wref] -> prediction1/8(wref)
  Delay2/1 -> prediction1/1(M2_iqref_prev)
  [M2_Speed_Error] -> Delay5/1
  Gain4/1 -> prediction1/13(ElectricalAngle)
  prediction1/7(M2_Speed_Error) -> [M2_Speed_Error]
  prediction1/1(M2_DutyA) -> [M2_DutyA]
  Delay5/1 -> prediction1/22(M2_Speed_Error_prev)
  [wmech_lowrate] -> Delay6/1
  [M2_iqs] -> prediction1/4(M2_IqMeasured)
  Delay18/1 -> prediction1/21(M2_IqRipplePrediction_prev)
  [M2_DutyC] -> Delay4/1
  [M2_ids] -> prediction1/3(M2_IdMeasured)
  prediction/6(M1_iqref) -> [M1_iqref]
  prediction1/6(M2_iqref) -> [M2_iqref]
  [M2_iqref] -> Delay2/1
  [M1_iqref] -> Delay/1
  connections:
  DCLINK_Cap/LConn1 -- Current Measurement/LConn1 -- Voltage Measurement3/LConn1
  Controlled Voltage Source/RConn1 -- Rin/RConn1
  Current Measurement3/RConn1 -- Permanent Magnet Synchronous Machine/LConn4
  Permanent Magnet Synchronous Machine/LConn3 -- Current Measurement2/RConn1
  Permanent Magnet Synchronous Machine/LConn2 -- Current Measurement1/RConn1
  Current Measurement1/LConn1 -- Ideal Switch/RConn1 -- Series RLC Branch/RConn1
  Mechanical Subsystem/LConn1 -- Permanent Magnet Synchronous Machine/LConn1 -- Permanent Magnet Synchronous Machine1/LConn1
  Permanent Magnet Synchronous Machine1/LConn4 -- Current Measurement6/RConn1
  Current Measurement6/LConn1 -- Inverter2/LConn3 -- Voltage Measurement5/LConn2 -- Voltage Measurement6/LConn1
  Permanent Magnet Synchronous Machine1/LConn3 -- Current Measurement5/RConn1
  Current Measurement2/LConn1 -- Voltage Measurement1/LConn1 -- Voltage Measurement/LConn2 -- Inverter1/LConn2
  Current Measurement4/RConn1 -- Permanent Magnet Synchronous Machine1/LConn2
  Rin/LConn1 -- Current Measurement/RConn1 -- Inverter2/RConn1 -- Inverter1/RConn1
  Voltage Measurement2/LConn2 -- Ideal Switch/LConn1 -- Series RLC Branch/LConn1 -- Inverter1/LConn1 -- Voltage Measurement/LConn1
  DCLINK_Cap/RConn1 -- Controlled Voltage Source/LConn1 -- Voltage Measurement3/LConn2 -- Inverter2/RConn2 -- Inverter1/RConn2
  Current Measurement4/LConn1 -- Inverter2/LConn1 -- Voltage Measurement4/LConn1 -- Voltage Measurement6/LConn2
  Current Measurement5/LConn1 -- Inverter2/LConn2 -- Voltage Measurement5/LConn1 -- Voltage Measurement4/LConn2
  Voltage Measurement1/LConn2 -- Inverter1/LConn3 -- Voltage Measurement2/LConn1 -- Current Measurement3/LConn1

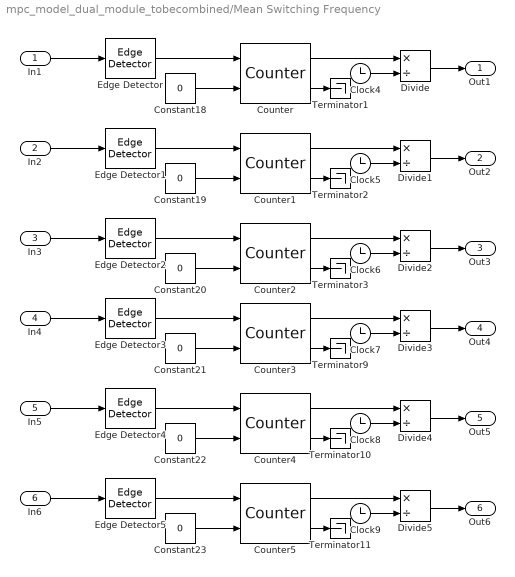
== system mpc_model_dual_module_tobecombined/Mean Switching Frequency ==
  In1 : Inport
  In2 : Inport  Port=2
  In3 : Inport  Port=3
  In4 : Inport  Port=4
  In5 : Inport  Port=5
  In6 : Inport  Port=6
  Clock{4..9} (6 alike) : Clock
  Constant{18..23} (6 alike) : Constant  Value=0
  Counter{,1..5} (6 alike) : dspswit3/Counter  Direction=Up  CountEvent=Rising edge  CounterSize=User defined  MaxCount=9999999999999999999  InitialCount=0  Output=Count and Hit  HitValue=32  ResetInput=on  SamplesPerFrame=1  Ts=1  CntDtype=double  HitDtype=Logical
  Divide{,1..5} (6 alike) : Product  Inputs=*/
  Edge Detector{,1..5} (6 alike) : dspswit3/Edge Detector  InputProcessing=Columns as channels (frame based)
      settings: SourceProductName=DSP System Toolbox  SourceProductBaseCode=DS
  Terminator{1..3,9..11} (6 alike) : Terminator
  Out1 : Outport
  Out2 : Outport  Port=2
  Out3 : Outport  Port=3
  Out4 : Outport  Port=4
  Out5 : Outport  Port=5
  Out6 : Outport  Port=6
  wires:
  Counter5/2 -> Terminator11/1
  Divide2/1 -> Out3/1
  Clock8/1 -> Divide4/2
  Counter1/1 -> Divide1/1
  Constant22/1 -> Counter4/2
  Edge Detector5/1 -> Counter5/1
  Counter/2 -> Terminator1/1
  Edge Detector/1 -> Counter/1
  Counter5/1 -> Divide5/1
  Edge Detector2/1 -> Counter2/1
  Edge Detector4/1 -> Counter4/1
  Clock7/1 -> Divide3/2
  Counter4/2 -> Terminator10/1
  Constant19/1 -> Counter1/2
  Counter2/2 -> Terminator3/1
  Clock9/1 -> Divide5/2
  Constant20/1 -> Counter2/2
  Divide5/1 -> Out6/1
  Constant23/1 -> Counter5/2
  Edge Detector1/1 -> Counter1/1
  Counter4/1 -> Divide4/1
  Clock5/1 -> Divide1/2
  Counter3/2 -> Terminator9/1
  Counter2/1 -> Divide2/1
  Constant18/1 -> Counter/2
  In6/1 -> Edge Detector5/1
  Constant21/1 -> Counter3/2
  Counter3/1 -> Divide3/1
  Edge Detector3/1 -> Counter3/1
  Divide3/1 -> Out4/1
  Counter1/2 -> Terminator2/1
  In5/1 -> Edge Detector4/1
  Clock6/1 -> Divide2/2
  Divide/1 -> Out1/1
  Counter/1 -> Divide/1
  Clock4/1 -> Divide/2
  Divide4/1 -> Out5/1
  In4/1 -> Edge Detector3/1
  In2/1 -> Edge Detector1/1
  Divide1/1 -> Out2/1
  In3/1 -> Edge Detector2/1
  In1/1 -> Edge Detector/1

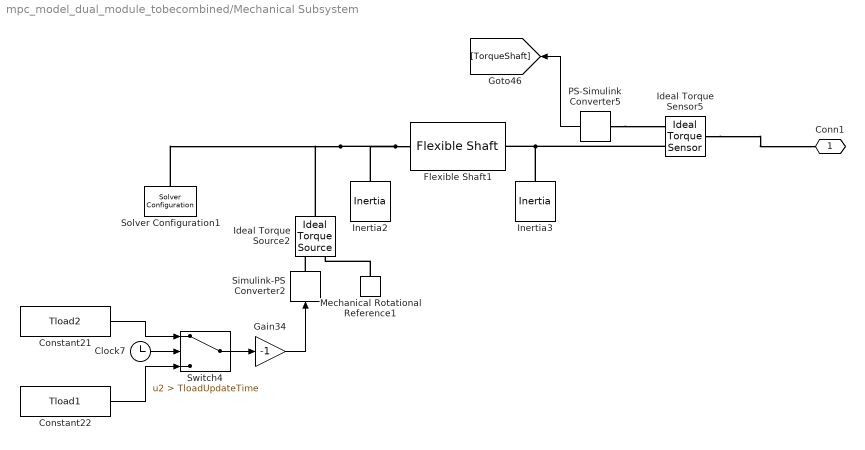
== system mpc_model_dual_module_tobecombined/Mechanical Subsystem ==
  Clock7 : Clock
  Constant21 : Constant  Value=Tload2
  Constant22 : Constant  Value=Tload1
  Flexible Shaft1 : sdl_lib/Couplings & Drives/Flexible Shaft  modelTransverse=simscape.enum.onoff.off  parameterization=1  n_segments=10  shaft_stiffness=MechanicalShaftStiffness N*m/rad  shaft_inertia=MechanicalShaftInertia kg*m^2  length=1 m  eiIN=5e5 m^4*Pa  rhoaIN=19 kg/m  shaft_construction=1  diameter_outer=0.075 m  diameter_inner=0.05 m  density=7.8e+3 kg/m^3  shear_modulus=7.93e+10 Pa  elastic_modulus=200e9 Pa  damping_ratio=MechanicalShaftDampingRatio  mu_visc=[ 0 0 ] N*m/(rad/s)  boundaryC=sdl.enum.shaftSupport.clamp  KtransC_row=[10000000, 10000000] N/m  KrotC_row=[10000000, 10000000] N*m/rad  boundaryR=sdl.enum.shaftSupport.clamp  KtransR_row=[10000000, 10000000] N/m  KrotR_row=[10000000, 10000000] N*m/rad  alpha=10 1/s  beta=1e-8 s  d_bearing_trans=[0, 0] N/(m/s)  d_bearing_rotation=[0, 0] N*m/(rad/s)  noDisk=sdl.enum.shaftDisks.none  zDisk=0.5 m  mDiskIN=2 kg  IdDiskIN=0.025 kg*m^2  IpDiskIN=0.050 kg*m^2  offsetMR=[.01, .01] m*kg  offsetMassLocation=[.33, .67] m  offsetMR_initialAngleIN=[0, pi] rad  AnalysisMethod=sdl.enum.bendingAnalysisMethod.LumpedMass  ModeInputMethod=sdl.enum.modeInputMethod.SimscapeDetermined  numModesIn=6  OmegaNom=100 rpm  dw=5 rad/s  dwRefineFactor=1e-4  wMax=50000 rad/s  dz=0.01 m  userMode_w=[162, 162, 649, 649, 1460, 1460, 2596, 2596] rad/s  userMode_z=[0 : 0.1 : 1] m  userMode_shape=[0, 0, 0, 0, 0, 0, 0, 0, 0, 0, 0, 0, 0, 0, 0, 0; .309, 0, 0, .309, .5878, 0, 0, .5878, .809, 0, 0, .809, .9511, 0, 0, .9511; .5878, 0, 0, .5878, .9511, 0, 0, .9511, .9511, 0, 0, .9511, .5878, 0, 0, .5878; .809, 0, 0, .809, .9511, 0, 0, .9511, .309, 0, 0, .309, -.5878, 0, 0, -.5878; .9511, 0, 0, .9511, .5878, 0, 0, .5878, -.5878, 0, 0, -.5878, -.9511, 0, 0, -.9511; 1, 0, 0, 1, 0, 0, 0, 0, -1, 0, 0, -1, 0, 0, 0, 0; .9511, 0, 0, .9511, -.5878, 0, 0, -.5878, -.5878, 0, 0, -.5878, .9511, 0, 0, .9511; .809, 0, 0, .809, -.9511, 0, 0, -.9511, .309, 0, 0, .309, .5878, 0, 0, .5878; .5878, 0, 0, .5878, -.9511, 0, 0, -.9511, .9511, 0, 0, .9511, -.5878, 0, 0, -.5878; .309, 0, 0, .309, -.5878, 0, 0, -.5878, .809, 0, 0, .809, -.9511, 0, 0, -.9511; 0, 0, 0, 0, 0, 0, 0, 0, 0, 0, 0, 0, 0, 0, 0, 0]  initial_deflection=0 rad  initial_velocity=0 rpm
      settings: SourceProductName=Simscape Driveline  SourceProductBaseCode=LD
  Gain34 : Gain  Gain=-1
  Ideal Torque Sensor5 : fl_lib/Mechanical/Mechanical Sensors/Ideal Torque Sensor
  Ideal Torque Source2 : fl_lib/Mechanical/Mechanical Sources/Ideal Torque Source
  Inertia2 : fl_lib/Mechanical/Rotational Elements/Inertia  inertia=MechanicalInertia1 kg*m^2  w_specify=off  w_priority=High  w=0 rad/s  w_nominal_specify=off  w_nominal_unit=rad/s  w_nominal_value=1  t_specify=off  t_priority=None  t=0 N*m  t_nominal_specify=off  t_nominal_unit=N*m  t_nominal_value=1
  Inertia3 : fl_lib/Mechanical/Rotational Elements/Inertia  inertia=MechanicalInertia1 kg*m^2  w_specify=off  w_priority=High  w=0 rad/s  w_nominal_specify=off  w_nominal_unit=rad/s  w_nominal_value=1  t_specify=off  t_priority=None  t=0 N*m  t_nominal_specify=off  t_nominal_unit=N*m  t_nominal_value=1
  Mechanical Rotational Reference1 : fl_lib/Mechanical/Rotational Elements/Mechanical Rotational Reference
  PS-Simulink Converter5 : nesl_utility/PS-Simulink Converter  PhysicalDomain=network_engine_domain  SubClassName=ps_output  LeftPortType=input  RightPortType=output  PseudoPeriodic=off  Frequencies=[]  Unit=1  AffineConversion=off
  Simulink-PS Converter2 : nesl_utility/Simulink-PS Converter  PhysicalDomain=network_engine_domain  SubClassName=ps_input  LeftPortType=input  RightPortType=output  PseudoPeriodic=off  Frequencies=[]  NoiseDistribution=none  NoiseParameters=[]  Unit=1  AffineConversion=off  FilteringAndDerivatives=zero  SimscapeFilterOrder=1  InputFilterTimeConstant=0.001  UdotUserProvided=1
  Solver Configuration1 : nesl_utility/Solver Configuration  PhysicalDomain=network_engine_domain  SubClassName=solver  LeftPortType=input  RightPortType=generic  Tones=[]  Harmonics=[]  SimulateNoise=off  Profile=off  UseLocalSampling=off  EnableSwitchedLinearOptims=on  FrequencyDomain=off  UseCCode=off  RelTol=0.001  AbsTol=1e-06  MinStep=1e-09  ToWorkspace=off  RevertToSquareIcSolve=off  NumHomotopyIterations=100  PhasorMode=off  PhasorModeNumHarmonics=1  DoDC=off  ResidualTolerance=1e-09  UseLocalSolver=off  LocalSolverChoice=NE_BACKWARD_EULER_ADVANCER  LocalSolverSampleTime=0.001  DoFixedCost=off  MaxNonlinIter=3  MaxModeIter=2  LinearAlgebra=Sparse  EquationFormulation=NE_TIME_EF  DelaysMemoryBudget=1024  AutomaticFiltering=on  FilteringTimeConstant=0.001  PartitionStorageMethod=AS_NEEDED  PartitionMemoryBudget=1024  PartitionMethod=FAST
  Switch4 : Switch  Criteria=u2 > Threshold  Threshold=TloadUpdateTime
  Conn1 : PMIOPort  Side=Left
  wires:
  Clock7/1 -> Switch4/2
  Constant21/1 -> Switch4/1
  Gain34/1 -> Simulink-PS Converter2/1
  PS-Simulink Converter5/1 -> [TorqueShaft]
  Switch4/1 -> Gain34/1
  Constant22/1 -> Switch4/3
  connections:
  Flexible Shaft1/LConn1 -- Inertia2/LConn1 -- Solver Configuration1/RConn1 -- Ideal Torque Source2/LConn1
  Ideal Torque Sensor5/LConn1 -- Conn1/RConn1
  Ideal Torque Sensor5/RConn1 -- Inertia3/LConn1 -- Flexible Shaft1/RConn1
  Simulink-PS Converter2/RConn1 -- Ideal Torque Source2/RConn1
  Mechanical Rotational Reference1/LConn1 -- Ideal Torque Source2/RConn2
  PS-Simulink Converter5/LConn1 -- Ideal Torque Sensor5/RConn2
